simulink model "PWM_STM32_g431xx_Boost_Converter"  (R2025b)
settings: Solver=FixedStepAuto  StartTime=0.0  StopTime=inf  FixedStep=Ts  RelTol=1e-3  EnableMultiTasking=on
InitFcn:
  | Startup_Parameters
values from neighbouring files (symbols this model uses):
  ARR = (Fclk/Dpwm) - 1    (= 339)    [Startup_Parameters.m]
  Ts = 1e-5    (= 1e-05)    [Startup_Parameters.m]    (also in Transfer_Functions_Boost_STM32.m = 2e-06)
  TsLED = 0.05    [Startup_Parameters.m]
libraries: stm32f4xxblockslib x4
settings Model: STM32="{\"DigitalPortWrite\":[{\"ID\":\"Blinky:1\"},{\"ID\":\"Blinky_Chidote:1\"},{\"ID\":\"PWM_STM32_g431xx:1\"},{\"ID\":\"PWM_STM32_g431xx_Boost_Converter:1\"},{\"ID\":\"PWM_STM32_g431xx_Boost_Converter:13\"}],\"PWMOutput\":[{\"ID\":\"Blinky_Chidote:3\"},{\"ID\":\"PWM_STM32_g431xx:3\"},{\"ID\":\"PWM_STM32_g431xx_Boost_Converter:3\"}],\"AnalogInput\":{\"ID\":\"PWM_STM32_g431xx_Boost_Converter:35\"}}"  Creator=Erick Negrete  LastModifiedBy=Erick Negrete
settings OptimizationCC: EnhancedBackFolding=on  PassReuseOutputArgsAs=Individual arguments  ZeroExternalMemoryAtStartup=off  ZeroInternalMemoryAtStartup=off  MaxStackSize=512  OptimizeBlockOrder=speed  DifferentSizesBufferReuse=on  OptimizationCustomize=off  EfficientTunableParamExpr=on
settings DebuggingCC: ParameterTunabilityLossMsg=error
settings HardwareCC: ProdBitPerPointer=32.0  ProdBitPerSizeT=32.0  ProdBitPerPtrDiffT=32.0  ProdLargestAtomicInteger=Long  ProdLargestAtomicFloat=Double  ProdWordSize=32.0  ProdLongLongMode=on  ProdHWDeviceType=ARM Compatible->ARM Cortex-M
settings SFSimCC: MATLABDynamicMemAlloc=off
settings RTWCC: SystemTargetFile=ert.tlc  HardwareBoard=STM32G4xx Based  TemplateMakefile=ert_default_tmf  Toolchain=GNU Tools for ARM Embedded Processors  IncludeHyperlinkInReport=on  Description=Embedded Coder
settings CodeAppCC: ForceParamTrailComments=on  IgnoreCustomStorageClasses=off  OperatorAnnotations=on  SimulinkDataObjDesc=on  SFDataObjDesc=on  InsertBlockDesc=on
settings ERTTargetCC: ExtModeTransport=3.0  ExtModeStaticAlloc=on  ExtModeStaticAllocSize=10000.0  ExtModeMexFile=ext_xcp  ExtModeIntrfLevel=Level2 - Open  InlinedParameterPlacement=Hierarchical  TargetLangStandard=C99 (ISO)  CodeReplacementLibrary=ARM Cortex-M

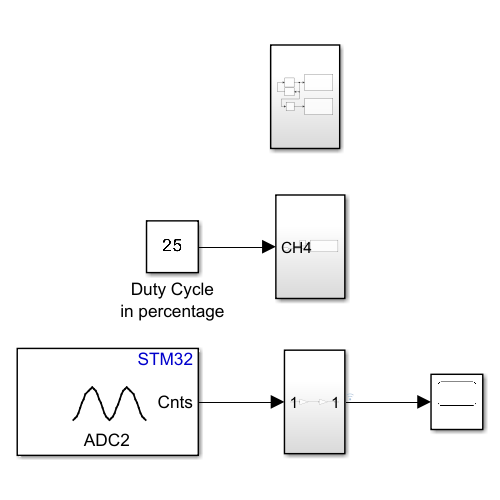
[thumbnail: Simulink's stored preview of the top-level diagram]
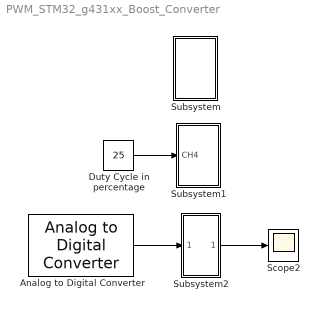
== system PWM_STM32_g431xx_Boost_Converter ==
  Analog to Digital Converter : stm32f4xxblockslib/Analog to Digital Converter  ADCModule=ADC2  ConversionGroup=Regular  TriggerMode=Trigger and read  NumberOfConversions=1  EnableBufferConv=off  BufferLength=1  OutputStatus=off  SampleTime=Ts  EnableSimPort=off  hoistedMaskSrc=ECSoC/ECSimCodegen/Analog to Digital Converter
  Duty Cycle in percentage : Constant  Value=25
  Scope2 : Scope
      settings: ActiveDisplayYMinimum=23.550602793693542  ActiveDisplayYMaximum=23.620107769966125
  Subsystem : Subsystem
  Subsystem1 : Subsystem
  Subsystem2 : Subsystem
  wires:
  Duty Cycle in percentage/1 -> Subsystem1/1(CH4)
  Analog to Digital Converter/1 -> Subsystem2/1(In1)
  Subsystem2/1(Out1) -> Scope2/1

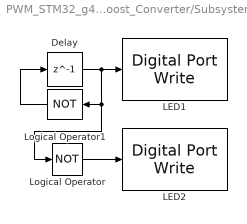
== system PWM_STM32_g431xx_Boost_Converter/Subsystem ==
  Delay : Delay  DelayLength=1  SampleTime=TsLED
  LED1 : stm32f4xxblockslib/Digital Port Write  PortName=GPIOB  PinNumber=[6]  ReadOperation=off  IOAsArray=on  EnableSimPort=off  hoistedMaskSrc=ECSoC/ECSimCodegen/Digital Port Write
      settings: LibrarySourceBlock=stm32g4xxblockslib/Digital Port Write
  LED2 : stm32f4xxblockslib/Digital Port Write  PortName=GPIOB  PinNumber=[5]  ReadOperation=off  IOAsArray=on  EnableSimPort=off  hoistedMaskSrc=ECSoC/ECSimCodegen/Digital Port Write
      settings: LibrarySourceBlock=stm32g4xxblockslib/Digital Port Write
  Logical Operator : Logic  Operator=NOT  AllPortsSameDT=off  OutDataTypeStr=boolean
  Logical Operator1 : Logic  Operator=NOT  AllPortsSameDT=off  OutDataTypeStr=boolean
  wires:
  Logical Operator/1 -> LED2/1
  Logical Operator1/1 -> Delay/1
  Delay/1 -> Logical Operator1/1, Logical Operator/1, LED1/1

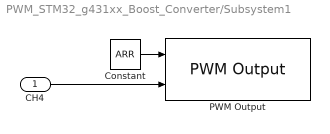
== system PWM_STM32_g431xx_Boost_Converter/Subsystem1 ==
  CH4 : Inport
  Constant : Constant  Value=ARR
  PWM Output : stm32f4xxblockslib/PWM Output  ProcessorFamily=STM32G4  TimerModule=TIM15  DutycycleUnits=Percentage  EnableChannel1=off  EnableCaptureCompare1Input=off  EnableCaptureCompare1ComplementaryInput=off  EnableOutputCompare1ModeInput=off  EnableChannel2=on  EnableCaptureCompare2Input=off  EnableCaptureCompare2ComplementaryInput=off  EnableOutputCompare2ModeInput=off  EnableChannel3=off  EnableCaptureCompare3Input=off  EnableCaptureCompare3ComplementaryInput=off  EnableOutputCompare3ModeInput=off  EnableChannel4=on  EnableCaptureCompare4Input=off  EnableCaptureCompare4ComplementaryInput=off  EnableOutputCompare4ModeInput=off  EnableChannel5=off  EnableCaptureCompare5Input=off  EnableOutputCompare5ModeInput=off  EnableChannel6=off  EnableCaptureCompare6Input=off  EnableOutputCompare6ModeInput=off  EnableCounterInput=off  EnableMainOutputInput=off  EnableFrequencyInput=on  SetRCAfterCE=off  OutputDirection=off  OutputMainOutputEnableStatus=off  SampleTime=0.1  EnableSimPort=off  EnableUpdateEvent=off  EnableCaptureCompare1Event=off  EnableCaptureCompare2Event=off  EnableCaptureCompare3Event=off  EnableCaptureCompare4Event=off  EnableTriggerEvent=off  EnableBreakEvent=off  EnableBreakEvent2=off  hoistedMaskSrc=ECSoC/ECSimCodegen/PWM Output
      settings: LibrarySourceBlock=stm32g4xxblockslib/PWM Output
  wires:
  Constant/1 -> PWM Output/1
  CH4/1 -> PWM Output/2

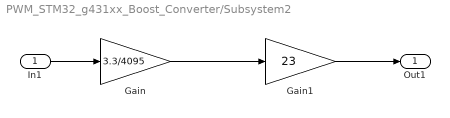
== system PWM_STM32_g431xx_Boost_Converter/Subsystem2 ==
  In1 : Inport
  Gain : Gain  Gain=3.3/4095
  Gain1 : Gain  Gain=23
  Out1 : Outport
  wires:
  In1/1 -> Gain/1
  Gain/1 -> Gain1/1
  Gain1/1 -> Out1/1
